simulink model "gm_UZ_EnDat"  (R2023b)
settings: Solver=FixedStepDiscrete  StartTime=0  StopTime=0.002  RelTol=1e-3
model workspace (MAT data in the model file):
  Select = 0
libraries: hdlsllib x314, hdlmdlgenlib x10, simulink x7, simulink_extras x3
(part 7 of 7)

== system gm_UZ_EnDat/UZ_ENDAT/ManualSerialize/padder/nibblepadding22/padding1 ==
  in : Inport  OutDataTypeStr=fixdt(0, 64, 0)  PortDimensions=1  SampleTime=1e-08
  Bit Shift2 : hdlsllib/Logic and Bit Operations/Bit Shift  mode=Shift Right Logical  N=double(1)
  Bit Slice2 : hdlsllib/Logic and Bit Operations/Bit Slice  lidx=double(0)  ridx=double(0)
  Data Type Conversion2 : DataTypeConversion  OutDataTypeStr=boolean  RndMeth=Nearest  SampleTime=1e-08  SaturateOnIntegerOverflow=off
  Switch2 : Switch  Criteria=u2 > Threshold  Threshold=double(0)  OutDataTypeStr=fixdt(0, 64, 0)  SampleTime=1e-08  SaturateOnIntegerOverflow=off  InputSameDT=off
  out : Outport  SampleTime=1e-08
  wires:
  Switch2/1 -> out/1
  Data Type Conversion2/1 -> Switch2/2
  Bit Slice2/1 -> Data Type Conversion2/1
  Bit Shift2/1 -> Switch2/3
  in/1 -> Bit Shift2/1, Bit Slice2/1, Switch2/1

== system gm_UZ_EnDat/UZ_ENDAT/ManualSerialize/padder/nibblepadding22/padding2 ==
  in : Inport  OutDataTypeStr=fixdt(0, 64, 0)  PortDimensions=1  SampleTime=1e-08
  Bit Shift2 : hdlsllib/Logic and Bit Operations/Bit Shift  mode=Shift Right Logical  N=double(1)
  Bit Slice2 : hdlsllib/Logic and Bit Operations/Bit Slice  lidx=double(0)  ridx=double(0)
  Data Type Conversion2 : DataTypeConversion  OutDataTypeStr=boolean  RndMeth=Nearest  SampleTime=1e-08  SaturateOnIntegerOverflow=off
  Switch2 : Switch  Criteria=u2 > Threshold  Threshold=double(0)  OutDataTypeStr=fixdt(0, 64, 0)  SampleTime=1e-08  SaturateOnIntegerOverflow=off  InputSameDT=off
  out : Outport  SampleTime=1e-08
  wires:
  in/1 -> Switch2/1, Bit Slice2/1, Bit Shift2/1
  Bit Shift2/1 -> Switch2/3
  Bit Slice2/1 -> Data Type Conversion2/1
  Data Type Conversion2/1 -> Switch2/2
  Switch2/1 -> out/1

== system gm_UZ_EnDat/UZ_ENDAT/ManualSerialize/padder/nibblepadding22/padding3 ==
  in : Inport  OutDataTypeStr=fixdt(0, 64, 0)  PortDimensions=1  SampleTime=1e-08
  Bit Shift2 : hdlsllib/Logic and Bit Operations/Bit Shift  mode=Shift Right Logical  N=double(1)
  Bit Slice2 : hdlsllib/Logic and Bit Operations/Bit Slice  lidx=double(0)  ridx=double(0)
  Data Type Conversion2 : DataTypeConversion  OutDataTypeStr=boolean  RndMeth=Nearest  SampleTime=1e-08  SaturateOnIntegerOverflow=off
  Switch2 : Switch  Criteria=u2 > Threshold  Threshold=double(0)  OutDataTypeStr=fixdt(0, 64, 0)  SampleTime=1e-08  SaturateOnIntegerOverflow=off  InputSameDT=off
  out : Outport  SampleTime=1e-08
  wires:
  in/1 -> Switch2/1, Bit Slice2/1, Bit Shift2/1
  Bit Shift2/1 -> Switch2/3
  Bit Slice2/1 -> Data Type Conversion2/1
  Data Type Conversion2/1 -> Switch2/2
  Switch2/1 -> out/1

== system gm_UZ_EnDat/UZ_ENDAT/ManualSerialize/padder/nibblepadding23/padding1 ==
  in : Inport  OutDataTypeStr=fixdt(0, 64, 0)  PortDimensions=1  SampleTime=1e-08
  Bit Shift2 : hdlsllib/Logic and Bit Operations/Bit Shift  mode=Shift Right Logical  N=double(1)
  Bit Slice2 : hdlsllib/Logic and Bit Operations/Bit Slice  lidx=double(0)  ridx=double(0)
  Data Type Conversion2 : DataTypeConversion  OutDataTypeStr=boolean  RndMeth=Nearest  SampleTime=1e-08  SaturateOnIntegerOverflow=off
  Switch2 : Switch  Criteria=u2 > Threshold  Threshold=double(0)  OutDataTypeStr=fixdt(0, 64, 0)  SampleTime=1e-08  SaturateOnIntegerOverflow=off  InputSameDT=off
  out : Outport  SampleTime=1e-08
  wires:
  Switch2/1 -> out/1
  Data Type Conversion2/1 -> Switch2/2
  Bit Slice2/1 -> Data Type Conversion2/1
  Bit Shift2/1 -> Switch2/3
  in/1 -> Bit Shift2/1, Bit Slice2/1, Switch2/1

== system gm_UZ_EnDat/UZ_ENDAT/ManualSerialize/padder/nibblepadding23/padding2 ==
  in : Inport  OutDataTypeStr=fixdt(0, 64, 0)  PortDimensions=1  SampleTime=1e-08
  Bit Shift2 : hdlsllib/Logic and Bit Operations/Bit Shift  mode=Shift Right Logical  N=double(1)
  Bit Slice2 : hdlsllib/Logic and Bit Operations/Bit Slice  lidx=double(0)  ridx=double(0)
  Data Type Conversion2 : DataTypeConversion  OutDataTypeStr=boolean  RndMeth=Nearest  SampleTime=1e-08  SaturateOnIntegerOverflow=off
  Switch2 : Switch  Criteria=u2 > Threshold  Threshold=double(0)  OutDataTypeStr=fixdt(0, 64, 0)  SampleTime=1e-08  SaturateOnIntegerOverflow=off  InputSameDT=off
  out : Outport  SampleTime=1e-08
  wires:
  in/1 -> Switch2/1, Bit Slice2/1, Bit Shift2/1
  Bit Shift2/1 -> Switch2/3
  Bit Slice2/1 -> Data Type Conversion2/1
  Data Type Conversion2/1 -> Switch2/2
  Switch2/1 -> out/1

== system gm_UZ_EnDat/UZ_ENDAT/ManualSerialize/padder/nibblepadding23/padding3 ==
  in : Inport  OutDataTypeStr=fixdt(0, 64, 0)  PortDimensions=1  SampleTime=1e-08
  Bit Shift2 : hdlsllib/Logic and Bit Operations/Bit Shift  mode=Shift Right Logical  N=double(1)
  Bit Slice2 : hdlsllib/Logic and Bit Operations/Bit Slice  lidx=double(0)  ridx=double(0)
  Data Type Conversion2 : DataTypeConversion  OutDataTypeStr=boolean  RndMeth=Nearest  SampleTime=1e-08  SaturateOnIntegerOverflow=off
  Switch2 : Switch  Criteria=u2 > Threshold  Threshold=double(0)  OutDataTypeStr=fixdt(0, 64, 0)  SampleTime=1e-08  SaturateOnIntegerOverflow=off  InputSameDT=off
  out : Outport  SampleTime=1e-08
  wires:
  in/1 -> Switch2/1, Bit Slice2/1, Bit Shift2/1
  Bit Shift2/1 -> Switch2/3
  Bit Slice2/1 -> Data Type Conversion2/1
  Data Type Conversion2/1 -> Switch2/2
  Switch2/1 -> out/1

== system gm_UZ_EnDat/UZ_ENDAT/ManualSerialize/padder/nibblepadding24/padding1 ==
  in : Inport  OutDataTypeStr=fixdt(0, 64, 0)  PortDimensions=1  SampleTime=1e-08
  Bit Shift2 : hdlsllib/Logic and Bit Operations/Bit Shift  mode=Shift Right Logical  N=double(1)
  Bit Slice2 : hdlsllib/Logic and Bit Operations/Bit Slice  lidx=double(0)  ridx=double(0)
  Data Type Conversion2 : DataTypeConversion  OutDataTypeStr=boolean  RndMeth=Nearest  SampleTime=1e-08  SaturateOnIntegerOverflow=off
  Switch2 : Switch  Criteria=u2 > Threshold  Threshold=double(0)  OutDataTypeStr=fixdt(0, 64, 0)  SampleTime=1e-08  SaturateOnIntegerOverflow=off  InputSameDT=off
  out : Outport  SampleTime=1e-08
  wires:
  Switch2/1 -> out/1
  Data Type Conversion2/1 -> Switch2/2
  Bit Slice2/1 -> Data Type Conversion2/1
  Bit Shift2/1 -> Switch2/3
  in/1 -> Bit Shift2/1, Bit Slice2/1, Switch2/1

== system gm_UZ_EnDat/UZ_ENDAT/ManualSerialize/padder/nibblepadding24/padding2 ==
  in : Inport  OutDataTypeStr=fixdt(0, 64, 0)  PortDimensions=1  SampleTime=1e-08
  Bit Shift2 : hdlsllib/Logic and Bit Operations/Bit Shift  mode=Shift Right Logical  N=double(1)
  Bit Slice2 : hdlsllib/Logic and Bit Operations/Bit Slice  lidx=double(0)  ridx=double(0)
  Data Type Conversion2 : DataTypeConversion  OutDataTypeStr=boolean  RndMeth=Nearest  SampleTime=1e-08  SaturateOnIntegerOverflow=off
  Switch2 : Switch  Criteria=u2 > Threshold  Threshold=double(0)  OutDataTypeStr=fixdt(0, 64, 0)  SampleTime=1e-08  SaturateOnIntegerOverflow=off  InputSameDT=off
  out : Outport  SampleTime=1e-08
  wires:
  in/1 -> Switch2/1, Bit Slice2/1, Bit Shift2/1
  Bit Shift2/1 -> Switch2/3
  Bit Slice2/1 -> Data Type Conversion2/1
  Data Type Conversion2/1 -> Switch2/2
  Switch2/1 -> out/1

== system gm_UZ_EnDat/UZ_ENDAT/ManualSerialize/padder/nibblepadding24/padding3 ==
  in : Inport  OutDataTypeStr=fixdt(0, 64, 0)  PortDimensions=1  SampleTime=1e-08
  Bit Shift2 : hdlsllib/Logic and Bit Operations/Bit Shift  mode=Shift Right Logical  N=double(1)
  Bit Slice2 : hdlsllib/Logic and Bit Operations/Bit Slice  lidx=double(0)  ridx=double(0)
  Data Type Conversion2 : DataTypeConversion  OutDataTypeStr=boolean  RndMeth=Nearest  SampleTime=1e-08  SaturateOnIntegerOverflow=off
  Switch2 : Switch  Criteria=u2 > Threshold  Threshold=double(0)  OutDataTypeStr=fixdt(0, 64, 0)  SampleTime=1e-08  SaturateOnIntegerOverflow=off  InputSameDT=off
  out : Outport  SampleTime=1e-08
  wires:
  in/1 -> Switch2/1, Bit Slice2/1, Bit Shift2/1
  Bit Shift2/1 -> Switch2/3
  Bit Slice2/1 -> Data Type Conversion2/1
  Data Type Conversion2/1 -> Switch2/2
  Switch2/1 -> out/1

== system gm_UZ_EnDat/UZ_ENDAT/ManualSerialize/padder/nibblepadding25/padding1 ==
  in : Inport  OutDataTypeStr=fixdt(0, 64, 0)  PortDimensions=1  SampleTime=1e-08
  Bit Shift2 : hdlsllib/Logic and Bit Operations/Bit Shift  mode=Shift Right Logical  N=double(1)
  Bit Slice2 : hdlsllib/Logic and Bit Operations/Bit Slice  lidx=double(0)  ridx=double(0)
  Data Type Conversion2 : DataTypeConversion  OutDataTypeStr=boolean  RndMeth=Nearest  SampleTime=1e-08  SaturateOnIntegerOverflow=off
  Switch2 : Switch  Criteria=u2 > Threshold  Threshold=double(0)  OutDataTypeStr=fixdt(0, 64, 0)  SampleTime=1e-08  SaturateOnIntegerOverflow=off  InputSameDT=off
  out : Outport  SampleTime=1e-08
  wires:
  Switch2/1 -> out/1
  Data Type Conversion2/1 -> Switch2/2
  Bit Slice2/1 -> Data Type Conversion2/1
  Bit Shift2/1 -> Switch2/3
  in/1 -> Bit Shift2/1, Bit Slice2/1, Switch2/1

== system gm_UZ_EnDat/UZ_ENDAT/ManualSerialize/padder/nibblepadding25/padding2 ==
  in : Inport  OutDataTypeStr=fixdt(0, 64, 0)  PortDimensions=1  SampleTime=1e-08
  Bit Shift2 : hdlsllib/Logic and Bit Operations/Bit Shift  mode=Shift Right Logical  N=double(1)
  Bit Slice2 : hdlsllib/Logic and Bit Operations/Bit Slice  lidx=double(0)  ridx=double(0)
  Data Type Conversion2 : DataTypeConversion  OutDataTypeStr=boolean  RndMeth=Nearest  SampleTime=1e-08  SaturateOnIntegerOverflow=off
  Switch2 : Switch  Criteria=u2 > Threshold  Threshold=double(0)  OutDataTypeStr=fixdt(0, 64, 0)  SampleTime=1e-08  SaturateOnIntegerOverflow=off  InputSameDT=off
  out : Outport  SampleTime=1e-08
  wires:
  in/1 -> Switch2/1, Bit Slice2/1, Bit Shift2/1
  Bit Shift2/1 -> Switch2/3
  Bit Slice2/1 -> Data Type Conversion2/1
  Data Type Conversion2/1 -> Switch2/2
  Switch2/1 -> out/1

== system gm_UZ_EnDat/UZ_ENDAT/ManualSerialize/padder/nibblepadding25/padding3 ==
  in : Inport  OutDataTypeStr=fixdt(0, 64, 0)  PortDimensions=1  SampleTime=1e-08
  Bit Shift2 : hdlsllib/Logic and Bit Operations/Bit Shift  mode=Shift Right Logical  N=double(1)
  Bit Slice2 : hdlsllib/Logic and Bit Operations/Bit Slice  lidx=double(0)  ridx=double(0)
  Data Type Conversion2 : DataTypeConversion  OutDataTypeStr=boolean  RndMeth=Nearest  SampleTime=1e-08  SaturateOnIntegerOverflow=off
  Switch2 : Switch  Criteria=u2 > Threshold  Threshold=double(0)  OutDataTypeStr=fixdt(0, 64, 0)  SampleTime=1e-08  SaturateOnIntegerOverflow=off  InputSameDT=off
  out : Outport  SampleTime=1e-08
  wires:
  in/1 -> Switch2/1, Bit Slice2/1, Bit Shift2/1
  Bit Shift2/1 -> Switch2/3
  Bit Slice2/1 -> Data Type Conversion2/1
  Data Type Conversion2/1 -> Switch2/2
  Switch2/1 -> out/1

== system gm_UZ_EnDat/UZ_ENDAT/ManualSerialize/padder/nibblepadding26/padding1 ==
  in : Inport  OutDataTypeStr=fixdt(0, 64, 0)  PortDimensions=1  SampleTime=1e-08
  Bit Shift2 : hdlsllib/Logic and Bit Operations/Bit Shift  mode=Shift Right Logical  N=double(1)
  Bit Slice2 : hdlsllib/Logic and Bit Operations/Bit Slice  lidx=double(0)  ridx=double(0)
  Data Type Conversion2 : DataTypeConversion  OutDataTypeStr=boolean  RndMeth=Nearest  SampleTime=1e-08  SaturateOnIntegerOverflow=off
  Switch2 : Switch  Criteria=u2 > Threshold  Threshold=double(0)  OutDataTypeStr=fixdt(0, 64, 0)  SampleTime=1e-08  SaturateOnIntegerOverflow=off  InputSameDT=off
  out : Outport  SampleTime=1e-08
  wires:
  Switch2/1 -> out/1
  Data Type Conversion2/1 -> Switch2/2
  Bit Slice2/1 -> Data Type Conversion2/1
  Bit Shift2/1 -> Switch2/3
  in/1 -> Bit Shift2/1, Bit Slice2/1, Switch2/1

== system gm_UZ_EnDat/UZ_ENDAT/ManualSerialize/padder/nibblepadding26/padding2 ==
  in : Inport  OutDataTypeStr=fixdt(0, 64, 0)  PortDimensions=1  SampleTime=1e-08
  Bit Shift2 : hdlsllib/Logic and Bit Operations/Bit Shift  mode=Shift Right Logical  N=double(1)
  Bit Slice2 : hdlsllib/Logic and Bit Operations/Bit Slice  lidx=double(0)  ridx=double(0)
  Data Type Conversion2 : DataTypeConversion  OutDataTypeStr=boolean  RndMeth=Nearest  SampleTime=1e-08  SaturateOnIntegerOverflow=off
  Switch2 : Switch  Criteria=u2 > Threshold  Threshold=double(0)  OutDataTypeStr=fixdt(0, 64, 0)  SampleTime=1e-08  SaturateOnIntegerOverflow=off  InputSameDT=off
  out : Outport  SampleTime=1e-08
  wires:
  in/1 -> Switch2/1, Bit Slice2/1, Bit Shift2/1
  Bit Shift2/1 -> Switch2/3
  Bit Slice2/1 -> Data Type Conversion2/1
  Data Type Conversion2/1 -> Switch2/2
  Switch2/1 -> out/1

== system gm_UZ_EnDat/UZ_ENDAT/ManualSerialize/padder/nibblepadding26/padding3 ==
  in : Inport  OutDataTypeStr=fixdt(0, 64, 0)  PortDimensions=1  SampleTime=1e-08
  Bit Shift2 : hdlsllib/Logic and Bit Operations/Bit Shift  mode=Shift Right Logical  N=double(1)
  Bit Slice2 : hdlsllib/Logic and Bit Operations/Bit Slice  lidx=double(0)  ridx=double(0)
  Data Type Conversion2 : DataTypeConversion  OutDataTypeStr=boolean  RndMeth=Nearest  SampleTime=1e-08  SaturateOnIntegerOverflow=off
  Switch2 : Switch  Criteria=u2 > Threshold  Threshold=double(0)  OutDataTypeStr=fixdt(0, 64, 0)  SampleTime=1e-08  SaturateOnIntegerOverflow=off  InputSameDT=off
  out : Outport  SampleTime=1e-08
  wires:
  in/1 -> Switch2/1, Bit Slice2/1, Bit Shift2/1
  Bit Shift2/1 -> Switch2/3
  Bit Slice2/1 -> Data Type Conversion2/1
  Data Type Conversion2/1 -> Switch2/2
  Switch2/1 -> out/1

== system gm_UZ_EnDat/UZ_ENDAT/ManualSerialize/padder/nibblepadding27/padding1 ==
  in : Inport  OutDataTypeStr=fixdt(0, 64, 0)  PortDimensions=1  SampleTime=1e-08
  Bit Shift2 : hdlsllib/Logic and Bit Operations/Bit Shift  mode=Shift Right Logical  N=double(1)
  Bit Slice2 : hdlsllib/Logic and Bit Operations/Bit Slice  lidx=double(0)  ridx=double(0)
  Data Type Conversion2 : DataTypeConversion  OutDataTypeStr=boolean  RndMeth=Nearest  SampleTime=1e-08  SaturateOnIntegerOverflow=off
  Switch2 : Switch  Criteria=u2 > Threshold  Threshold=double(0)  OutDataTypeStr=fixdt(0, 64, 0)  SampleTime=1e-08  SaturateOnIntegerOverflow=off  InputSameDT=off
  out : Outport  SampleTime=1e-08
  wires:
  Switch2/1 -> out/1
  Data Type Conversion2/1 -> Switch2/2
  Bit Slice2/1 -> Data Type Conversion2/1
  Bit Shift2/1 -> Switch2/3
  in/1 -> Bit Shift2/1, Bit Slice2/1, Switch2/1

== system gm_UZ_EnDat/UZ_ENDAT/ManualSerialize/padder/nibblepadding27/padding2 ==
  in : Inport  OutDataTypeStr=fixdt(0, 64, 0)  PortDimensions=1  SampleTime=1e-08
  Bit Shift2 : hdlsllib/Logic and Bit Operations/Bit Shift  mode=Shift Right Logical  N=double(1)
  Bit Slice2 : hdlsllib/Logic and Bit Operations/Bit Slice  lidx=double(0)  ridx=double(0)
  Data Type Conversion2 : DataTypeConversion  OutDataTypeStr=boolean  RndMeth=Nearest  SampleTime=1e-08  SaturateOnIntegerOverflow=off
  Switch2 : Switch  Criteria=u2 > Threshold  Threshold=double(0)  OutDataTypeStr=fixdt(0, 64, 0)  SampleTime=1e-08  SaturateOnIntegerOverflow=off  InputSameDT=off
  out : Outport  SampleTime=1e-08
  wires:
  in/1 -> Switch2/1, Bit Slice2/1, Bit Shift2/1
  Bit Shift2/1 -> Switch2/3
  Bit Slice2/1 -> Data Type Conversion2/1
  Data Type Conversion2/1 -> Switch2/2
  Switch2/1 -> out/1

== system gm_UZ_EnDat/UZ_ENDAT/ManualSerialize/padder/nibblepadding27/padding3 ==
  in : Inport  OutDataTypeStr=fixdt(0, 64, 0)  PortDimensions=1  SampleTime=1e-08
  Bit Shift2 : hdlsllib/Logic and Bit Operations/Bit Shift  mode=Shift Right Logical  N=double(1)
  Bit Slice2 : hdlsllib/Logic and Bit Operations/Bit Slice  lidx=double(0)  ridx=double(0)
  Data Type Conversion2 : DataTypeConversion  OutDataTypeStr=boolean  RndMeth=Nearest  SampleTime=1e-08  SaturateOnIntegerOverflow=off
  Switch2 : Switch  Criteria=u2 > Threshold  Threshold=double(0)  OutDataTypeStr=fixdt(0, 64, 0)  SampleTime=1e-08  SaturateOnIntegerOverflow=off  InputSameDT=off
  out : Outport  SampleTime=1e-08
  wires:
  in/1 -> Switch2/1, Bit Slice2/1, Bit Shift2/1
  Bit Shift2/1 -> Switch2/3
  Bit Slice2/1 -> Data Type Conversion2/1
  Data Type Conversion2/1 -> Switch2/2
  Switch2/1 -> out/1

== system gm_UZ_EnDat/UZ_ENDAT/ManualSerialize/padder/nibblepadding28/padding1 ==
  in : Inport  OutDataTypeStr=fixdt(0, 64, 0)  PortDimensions=1  SampleTime=1e-08
  Bit Shift2 : hdlsllib/Logic and Bit Operations/Bit Shift  mode=Shift Right Logical  N=double(1)
  Bit Slice2 : hdlsllib/Logic and Bit Operations/Bit Slice  lidx=double(0)  ridx=double(0)
  Data Type Conversion2 : DataTypeConversion  OutDataTypeStr=boolean  RndMeth=Nearest  SampleTime=1e-08  SaturateOnIntegerOverflow=off
  Switch2 : Switch  Criteria=u2 > Threshold  Threshold=double(0)  OutDataTypeStr=fixdt(0, 64, 0)  SampleTime=1e-08  SaturateOnIntegerOverflow=off  InputSameDT=off
  out : Outport  SampleTime=1e-08
  wires:
  Switch2/1 -> out/1
  Data Type Conversion2/1 -> Switch2/2
  Bit Slice2/1 -> Data Type Conversion2/1
  Bit Shift2/1 -> Switch2/3
  in/1 -> Bit Shift2/1, Bit Slice2/1, Switch2/1

== system gm_UZ_EnDat/UZ_ENDAT/ManualSerialize/padder/nibblepadding28/padding2 ==
  in : Inport  OutDataTypeStr=fixdt(0, 64, 0)  PortDimensions=1  SampleTime=1e-08
  Bit Shift2 : hdlsllib/Logic and Bit Operations/Bit Shift  mode=Shift Right Logical  N=double(1)
  Bit Slice2 : hdlsllib/Logic and Bit Operations/Bit Slice  lidx=double(0)  ridx=double(0)
  Data Type Conversion2 : DataTypeConversion  OutDataTypeStr=boolean  RndMeth=Nearest  SampleTime=1e-08  SaturateOnIntegerOverflow=off
  Switch2 : Switch  Criteria=u2 > Threshold  Threshold=double(0)  OutDataTypeStr=fixdt(0, 64, 0)  SampleTime=1e-08  SaturateOnIntegerOverflow=off  InputSameDT=off
  out : Outport  SampleTime=1e-08
  wires:
  in/1 -> Switch2/1, Bit Slice2/1, Bit Shift2/1
  Bit Shift2/1 -> Switch2/3
  Bit Slice2/1 -> Data Type Conversion2/1
  Data Type Conversion2/1 -> Switch2/2
  Switch2/1 -> out/1

== system gm_UZ_EnDat/UZ_ENDAT/ManualSerialize/padder/nibblepadding28/padding3 ==
  in : Inport  OutDataTypeStr=fixdt(0, 64, 0)  PortDimensions=1  SampleTime=1e-08
  Bit Shift2 : hdlsllib/Logic and Bit Operations/Bit Shift  mode=Shift Right Logical  N=double(1)
  Bit Slice2 : hdlsllib/Logic and Bit Operations/Bit Slice  lidx=double(0)  ridx=double(0)
  Data Type Conversion2 : DataTypeConversion  OutDataTypeStr=boolean  RndMeth=Nearest  SampleTime=1e-08  SaturateOnIntegerOverflow=off
  Switch2 : Switch  Criteria=u2 > Threshold  Threshold=double(0)  OutDataTypeStr=fixdt(0, 64, 0)  SampleTime=1e-08  SaturateOnIntegerOverflow=off  InputSameDT=off
  out : Outport  SampleTime=1e-08
  wires:
  in/1 -> Switch2/1, Bit Slice2/1, Bit Shift2/1
  Bit Shift2/1 -> Switch2/3
  Bit Slice2/1 -> Data Type Conversion2/1
  Data Type Conversion2/1 -> Switch2/2
  Switch2/1 -> out/1

== system gm_UZ_EnDat/UZ_ENDAT/ManualSerialize/padder/nibblepadding29/padding1 ==
  in : Inport  OutDataTypeStr=fixdt(0, 64, 0)  PortDimensions=1  SampleTime=1e-08
  Bit Shift2 : hdlsllib/Logic and Bit Operations/Bit Shift  mode=Shift Right Logical  N=double(1)
  Bit Slice2 : hdlsllib/Logic and Bit Operations/Bit Slice  lidx=double(0)  ridx=double(0)
  Data Type Conversion2 : DataTypeConversion  OutDataTypeStr=boolean  RndMeth=Nearest  SampleTime=1e-08  SaturateOnIntegerOverflow=off
  Switch2 : Switch  Criteria=u2 > Threshold  Threshold=double(0)  OutDataTypeStr=fixdt(0, 64, 0)  SampleTime=1e-08  SaturateOnIntegerOverflow=off  InputSameDT=off
  out : Outport  SampleTime=1e-08
  wires:
  Switch2/1 -> out/1
  Data Type Conversion2/1 -> Switch2/2
  Bit Slice2/1 -> Data Type Conversion2/1
  Bit Shift2/1 -> Switch2/3
  in/1 -> Bit Shift2/1, Bit Slice2/1, Switch2/1

== system gm_UZ_EnDat/UZ_ENDAT/ManualSerialize/padder/nibblepadding29/padding2 ==
  in : Inport  OutDataTypeStr=fixdt(0, 64, 0)  PortDimensions=1  SampleTime=1e-08
  Bit Shift2 : hdlsllib/Logic and Bit Operations/Bit Shift  mode=Shift Right Logical  N=double(1)
  Bit Slice2 : hdlsllib/Logic and Bit Operations/Bit Slice  lidx=double(0)  ridx=double(0)
  Data Type Conversion2 : DataTypeConversion  OutDataTypeStr=boolean  RndMeth=Nearest  SampleTime=1e-08  SaturateOnIntegerOverflow=off
  Switch2 : Switch  Criteria=u2 > Threshold  Threshold=double(0)  OutDataTypeStr=fixdt(0, 64, 0)  SampleTime=1e-08  SaturateOnIntegerOverflow=off  InputSameDT=off
  out : Outport  SampleTime=1e-08
  wires:
  in/1 -> Switch2/1, Bit Slice2/1, Bit Shift2/1
  Bit Shift2/1 -> Switch2/3
  Bit Slice2/1 -> Data Type Conversion2/1
  Data Type Conversion2/1 -> Switch2/2
  Switch2/1 -> out/1

== system gm_UZ_EnDat/UZ_ENDAT/ManualSerialize/padder/nibblepadding29/padding3 ==
  in : Inport  OutDataTypeStr=fixdt(0, 64, 0)  PortDimensions=1  SampleTime=1e-08
  Bit Shift2 : hdlsllib/Logic and Bit Operations/Bit Shift  mode=Shift Right Logical  N=double(1)
  Bit Slice2 : hdlsllib/Logic and Bit Operations/Bit Slice  lidx=double(0)  ridx=double(0)
  Data Type Conversion2 : DataTypeConversion  OutDataTypeStr=boolean  RndMeth=Nearest  SampleTime=1e-08  SaturateOnIntegerOverflow=off
  Switch2 : Switch  Criteria=u2 > Threshold  Threshold=double(0)  OutDataTypeStr=fixdt(0, 64, 0)  SampleTime=1e-08  SaturateOnIntegerOverflow=off  InputSameDT=off
  out : Outport  SampleTime=1e-08
  wires:
  in/1 -> Switch2/1, Bit Slice2/1, Bit Shift2/1
  Bit Shift2/1 -> Switch2/3
  Bit Slice2/1 -> Data Type Conversion2/1
  Data Type Conversion2/1 -> Switch2/2
  Switch2/1 -> out/1

== system gm_UZ_EnDat/UZ_ENDAT/ManualSerialize/padder/nibblepadding3/padding1 ==
  in : Inport  OutDataTypeStr=fixdt(0, 64, 0)  PortDimensions=1  SampleTime=1e-08
  Bit Shift2 : hdlsllib/Logic and Bit Operations/Bit Shift  mode=Shift Right Logical  N=double(1)
  Bit Slice2 : hdlsllib/Logic and Bit Operations/Bit Slice  lidx=double(0)  ridx=double(0)
  Data Type Conversion2 : DataTypeConversion  OutDataTypeStr=boolean  RndMeth=Nearest  SampleTime=1e-08  SaturateOnIntegerOverflow=off
  Switch2 : Switch  Criteria=u2 > Threshold  Threshold=double(0)  OutDataTypeStr=fixdt(0, 64, 0)  SampleTime=1e-08  SaturateOnIntegerOverflow=off  InputSameDT=off
  out : Outport  SampleTime=1e-08
  wires:
  Switch2/1 -> out/1
  Data Type Conversion2/1 -> Switch2/2
  Bit Slice2/1 -> Data Type Conversion2/1
  Bit Shift2/1 -> Switch2/3
  in/1 -> Bit Shift2/1, Bit Slice2/1, Switch2/1

== system gm_UZ_EnDat/UZ_ENDAT/ManualSerialize/padder/nibblepadding3/padding2 ==
  in : Inport  OutDataTypeStr=fixdt(0, 64, 0)  PortDimensions=1  SampleTime=1e-08
  Bit Shift2 : hdlsllib/Logic and Bit Operations/Bit Shift  mode=Shift Right Logical  N=double(1)
  Bit Slice2 : hdlsllib/Logic and Bit Operations/Bit Slice  lidx=double(0)  ridx=double(0)
  Data Type Conversion2 : DataTypeConversion  OutDataTypeStr=boolean  RndMeth=Nearest  SampleTime=1e-08  SaturateOnIntegerOverflow=off
  Switch2 : Switch  Criteria=u2 > Threshold  Threshold=double(0)  OutDataTypeStr=fixdt(0, 64, 0)  SampleTime=1e-08  SaturateOnIntegerOverflow=off  InputSameDT=off
  out : Outport  SampleTime=1e-08
  wires:
  in/1 -> Switch2/1, Bit Slice2/1, Bit Shift2/1
  Bit Shift2/1 -> Switch2/3
  Bit Slice2/1 -> Data Type Conversion2/1
  Data Type Conversion2/1 -> Switch2/2
  Switch2/1 -> out/1

== system gm_UZ_EnDat/UZ_ENDAT/ManualSerialize/padder/nibblepadding3/padding3 ==
  in : Inport  OutDataTypeStr=fixdt(0, 64, 0)  PortDimensions=1  SampleTime=1e-08
  Bit Shift2 : hdlsllib/Logic and Bit Operations/Bit Shift  mode=Shift Right Logical  N=double(1)
  Bit Slice2 : hdlsllib/Logic and Bit Operations/Bit Slice  lidx=double(0)  ridx=double(0)
  Data Type Conversion2 : DataTypeConversion  OutDataTypeStr=boolean  RndMeth=Nearest  SampleTime=1e-08  SaturateOnIntegerOverflow=off
  Switch2 : Switch  Criteria=u2 > Threshold  Threshold=double(0)  OutDataTypeStr=fixdt(0, 64, 0)  SampleTime=1e-08  SaturateOnIntegerOverflow=off  InputSameDT=off
  out : Outport  SampleTime=1e-08
  wires:
  in/1 -> Switch2/1, Bit Slice2/1, Bit Shift2/1
  Bit Shift2/1 -> Switch2/3
  Bit Slice2/1 -> Data Type Conversion2/1
  Data Type Conversion2/1 -> Switch2/2
  Switch2/1 -> out/1

== system gm_UZ_EnDat/UZ_ENDAT/ManualSerialize/padder/nibblepadding30/padding1 ==
  in : Inport  OutDataTypeStr=fixdt(0, 64, 0)  PortDimensions=1  SampleTime=1e-08
  Bit Shift2 : hdlsllib/Logic and Bit Operations/Bit Shift  mode=Shift Right Logical  N=double(1)
  Bit Slice2 : hdlsllib/Logic and Bit Operations/Bit Slice  lidx=double(0)  ridx=double(0)
  Data Type Conversion2 : DataTypeConversion  OutDataTypeStr=boolean  RndMeth=Nearest  SampleTime=1e-08  SaturateOnIntegerOverflow=off
  Switch2 : Switch  Criteria=u2 > Threshold  Threshold=double(0)  OutDataTypeStr=fixdt(0, 64, 0)  SampleTime=1e-08  SaturateOnIntegerOverflow=off  InputSameDT=off
  out : Outport  SampleTime=1e-08
  wires:
  Switch2/1 -> out/1
  Data Type Conversion2/1 -> Switch2/2
  Bit Slice2/1 -> Data Type Conversion2/1
  Bit Shift2/1 -> Switch2/3
  in/1 -> Bit Shift2/1, Bit Slice2/1, Switch2/1

== system gm_UZ_EnDat/UZ_ENDAT/ManualSerialize/padder/nibblepadding30/padding2 ==
  in : Inport  OutDataTypeStr=fixdt(0, 64, 0)  PortDimensions=1  SampleTime=1e-08
  Bit Shift2 : hdlsllib/Logic and Bit Operations/Bit Shift  mode=Shift Right Logical  N=double(1)
  Bit Slice2 : hdlsllib/Logic and Bit Operations/Bit Slice  lidx=double(0)  ridx=double(0)
  Data Type Conversion2 : DataTypeConversion  OutDataTypeStr=boolean  RndMeth=Nearest  SampleTime=1e-08  SaturateOnIntegerOverflow=off
  Switch2 : Switch  Criteria=u2 > Threshold  Threshold=double(0)  OutDataTypeStr=fixdt(0, 64, 0)  SampleTime=1e-08  SaturateOnIntegerOverflow=off  InputSameDT=off
  out : Outport  SampleTime=1e-08
  wires:
  in/1 -> Switch2/1, Bit Slice2/1, Bit Shift2/1
  Bit Shift2/1 -> Switch2/3
  Bit Slice2/1 -> Data Type Conversion2/1
  Data Type Conversion2/1 -> Switch2/2
  Switch2/1 -> out/1

== system gm_UZ_EnDat/UZ_ENDAT/ManualSerialize/padder/nibblepadding30/padding3 ==
  in : Inport  OutDataTypeStr=fixdt(0, 64, 0)  PortDimensions=1  SampleTime=1e-08
  Bit Shift2 : hdlsllib/Logic and Bit Operations/Bit Shift  mode=Shift Right Logical  N=double(1)
  Bit Slice2 : hdlsllib/Logic and Bit Operations/Bit Slice  lidx=double(0)  ridx=double(0)
  Data Type Conversion2 : DataTypeConversion  OutDataTypeStr=boolean  RndMeth=Nearest  SampleTime=1e-08  SaturateOnIntegerOverflow=off
  Switch2 : Switch  Criteria=u2 > Threshold  Threshold=double(0)  OutDataTypeStr=fixdt(0, 64, 0)  SampleTime=1e-08  SaturateOnIntegerOverflow=off  InputSameDT=off
  out : Outport  SampleTime=1e-08
  wires:
  in/1 -> Switch2/1, Bit Slice2/1, Bit Shift2/1
  Bit Shift2/1 -> Switch2/3
  Bit Slice2/1 -> Data Type Conversion2/1
  Data Type Conversion2/1 -> Switch2/2
  Switch2/1 -> out/1

== system gm_UZ_EnDat/UZ_ENDAT/ManualSerialize/padder/nibblepadding4/padding1 ==
  in : Inport  OutDataTypeStr=fixdt(0, 64, 0)  PortDimensions=1  SampleTime=1e-08
  Bit Shift2 : hdlsllib/Logic and Bit Operations/Bit Shift  mode=Shift Right Logical  N=double(1)
  Bit Slice2 : hdlsllib/Logic and Bit Operations/Bit Slice  lidx=double(0)  ridx=double(0)
  Data Type Conversion2 : DataTypeConversion  OutDataTypeStr=boolean  RndMeth=Nearest  SampleTime=1e-08  SaturateOnIntegerOverflow=off
  Switch2 : Switch  Criteria=u2 > Threshold  Threshold=double(0)  OutDataTypeStr=fixdt(0, 64, 0)  SampleTime=1e-08  SaturateOnIntegerOverflow=off  InputSameDT=off
  out : Outport  SampleTime=1e-08
  wires:
  Switch2/1 -> out/1
  Data Type Conversion2/1 -> Switch2/2
  Bit Slice2/1 -> Data Type Conversion2/1
  Bit Shift2/1 -> Switch2/3
  in/1 -> Bit Shift2/1, Bit Slice2/1, Switch2/1

== system gm_UZ_EnDat/UZ_ENDAT/ManualSerialize/padder/nibblepadding4/padding2 ==
  in : Inport  OutDataTypeStr=fixdt(0, 64, 0)  PortDimensions=1  SampleTime=1e-08
  Bit Shift2 : hdlsllib/Logic and Bit Operations/Bit Shift  mode=Shift Right Logical  N=double(1)
  Bit Slice2 : hdlsllib/Logic and Bit Operations/Bit Slice  lidx=double(0)  ridx=double(0)
  Data Type Conversion2 : DataTypeConversion  OutDataTypeStr=boolean  RndMeth=Nearest  SampleTime=1e-08  SaturateOnIntegerOverflow=off
  Switch2 : Switch  Criteria=u2 > Threshold  Threshold=double(0)  OutDataTypeStr=fixdt(0, 64, 0)  SampleTime=1e-08  SaturateOnIntegerOverflow=off  InputSameDT=off
  out : Outport  SampleTime=1e-08
  wires:
  in/1 -> Switch2/1, Bit Slice2/1, Bit Shift2/1
  Bit Shift2/1 -> Switch2/3
  Bit Slice2/1 -> Data Type Conversion2/1
  Data Type Conversion2/1 -> Switch2/2
  Switch2/1 -> out/1

== system gm_UZ_EnDat/UZ_ENDAT/ManualSerialize/padder/nibblepadding4/padding3 ==
  in : Inport  OutDataTypeStr=fixdt(0, 64, 0)  PortDimensions=1  SampleTime=1e-08
  Bit Shift2 : hdlsllib/Logic and Bit Operations/Bit Shift  mode=Shift Right Logical  N=double(1)
  Bit Slice2 : hdlsllib/Logic and Bit Operations/Bit Slice  lidx=double(0)  ridx=double(0)
  Data Type Conversion2 : DataTypeConversion  OutDataTypeStr=boolean  RndMeth=Nearest  SampleTime=1e-08  SaturateOnIntegerOverflow=off
  Switch2 : Switch  Criteria=u2 > Threshold  Threshold=double(0)  OutDataTypeStr=fixdt(0, 64, 0)  SampleTime=1e-08  SaturateOnIntegerOverflow=off  InputSameDT=off
  out : Outport  SampleTime=1e-08
  wires:
  in/1 -> Switch2/1, Bit Slice2/1, Bit Shift2/1
  Bit Shift2/1 -> Switch2/3
  Bit Slice2/1 -> Data Type Conversion2/1
  Data Type Conversion2/1 -> Switch2/2
  Switch2/1 -> out/1

== system gm_UZ_EnDat/UZ_ENDAT/ManualSerialize/padder/nibblepadding6/padding1 ==
  in : Inport  OutDataTypeStr=fixdt(0, 64, 0)  PortDimensions=1  SampleTime=1e-08
  Bit Shift2 : hdlsllib/Logic and Bit Operations/Bit Shift  mode=Shift Right Logical  N=double(1)
  Bit Slice2 : hdlsllib/Logic and Bit Operations/Bit Slice  lidx=double(0)  ridx=double(0)
  Data Type Conversion2 : DataTypeConversion  OutDataTypeStr=boolean  RndMeth=Nearest  SampleTime=1e-08  SaturateOnIntegerOverflow=off
  Switch2 : Switch  Criteria=u2 > Threshold  Threshold=double(0)  OutDataTypeStr=fixdt(0, 64, 0)  SampleTime=1e-08  SaturateOnIntegerOverflow=off  InputSameDT=off
  out : Outport  SampleTime=1e-08
  wires:
  Switch2/1 -> out/1
  Data Type Conversion2/1 -> Switch2/2
  Bit Slice2/1 -> Data Type Conversion2/1
  Bit Shift2/1 -> Switch2/3
  in/1 -> Bit Shift2/1, Bit Slice2/1, Switch2/1

== system gm_UZ_EnDat/UZ_ENDAT/ManualSerialize/padder/nibblepadding6/padding2 ==
  in : Inport  OutDataTypeStr=fixdt(0, 64, 0)  PortDimensions=1  SampleTime=1e-08
  Bit Shift2 : hdlsllib/Logic and Bit Operations/Bit Shift  mode=Shift Right Logical  N=double(1)
  Bit Slice2 : hdlsllib/Logic and Bit Operations/Bit Slice  lidx=double(0)  ridx=double(0)
  Data Type Conversion2 : DataTypeConversion  OutDataTypeStr=boolean  RndMeth=Nearest  SampleTime=1e-08  SaturateOnIntegerOverflow=off
  Switch2 : Switch  Criteria=u2 > Threshold  Threshold=double(0)  OutDataTypeStr=fixdt(0, 64, 0)  SampleTime=1e-08  SaturateOnIntegerOverflow=off  InputSameDT=off
  out : Outport  SampleTime=1e-08
  wires:
  in/1 -> Switch2/1, Bit Slice2/1, Bit Shift2/1
  Bit Shift2/1 -> Switch2/3
  Bit Slice2/1 -> Data Type Conversion2/1
  Data Type Conversion2/1 -> Switch2/2
  Switch2/1 -> out/1

== system gm_UZ_EnDat/UZ_ENDAT/ManualSerialize/padder/nibblepadding6/padding3 ==
  in : Inport  OutDataTypeStr=fixdt(0, 64, 0)  PortDimensions=1  SampleTime=1e-08
  Bit Shift2 : hdlsllib/Logic and Bit Operations/Bit Shift  mode=Shift Right Logical  N=double(1)
  Bit Slice2 : hdlsllib/Logic and Bit Operations/Bit Slice  lidx=double(0)  ridx=double(0)
  Data Type Conversion2 : DataTypeConversion  OutDataTypeStr=boolean  RndMeth=Nearest  SampleTime=1e-08  SaturateOnIntegerOverflow=off
  Switch2 : Switch  Criteria=u2 > Threshold  Threshold=double(0)  OutDataTypeStr=fixdt(0, 64, 0)  SampleTime=1e-08  SaturateOnIntegerOverflow=off  InputSameDT=off
  out : Outport  SampleTime=1e-08
  wires:
  in/1 -> Switch2/1, Bit Slice2/1, Bit Shift2/1
  Bit Shift2/1 -> Switch2/3
  Bit Slice2/1 -> Data Type Conversion2/1
  Data Type Conversion2/1 -> Switch2/2
  Switch2/1 -> out/1

== system gm_UZ_EnDat/UZ_ENDAT/ManualSerialize/padder/nibblepadding7/padding1 ==
  in : Inport  OutDataTypeStr=fixdt(0, 64, 0)  PortDimensions=1  SampleTime=1e-08
  Bit Shift2 : hdlsllib/Logic and Bit Operations/Bit Shift  mode=Shift Right Logical  N=double(1)
  Bit Slice2 : hdlsllib/Logic and Bit Operations/Bit Slice  lidx=double(0)  ridx=double(0)
  Data Type Conversion2 : DataTypeConversion  OutDataTypeStr=boolean  RndMeth=Nearest  SampleTime=1e-08  SaturateOnIntegerOverflow=off
  Switch2 : Switch  Criteria=u2 > Threshold  Threshold=double(0)  OutDataTypeStr=fixdt(0, 64, 0)  SampleTime=1e-08  SaturateOnIntegerOverflow=off  InputSameDT=off
  out : Outport  SampleTime=1e-08
  wires:
  Switch2/1 -> out/1
  Data Type Conversion2/1 -> Switch2/2
  Bit Slice2/1 -> Data Type Conversion2/1
  Bit Shift2/1 -> Switch2/3
  in/1 -> Bit Shift2/1, Bit Slice2/1, Switch2/1

== system gm_UZ_EnDat/UZ_ENDAT/ManualSerialize/padder/nibblepadding7/padding2 ==
  in : Inport  OutDataTypeStr=fixdt(0, 64, 0)  PortDimensions=1  SampleTime=1e-08
  Bit Shift2 : hdlsllib/Logic and Bit Operations/Bit Shift  mode=Shift Right Logical  N=double(1)
  Bit Slice2 : hdlsllib/Logic and Bit Operations/Bit Slice  lidx=double(0)  ridx=double(0)
  Data Type Conversion2 : DataTypeConversion  OutDataTypeStr=boolean  RndMeth=Nearest  SampleTime=1e-08  SaturateOnIntegerOverflow=off
  Switch2 : Switch  Criteria=u2 > Threshold  Threshold=double(0)  OutDataTypeStr=fixdt(0, 64, 0)  SampleTime=1e-08  SaturateOnIntegerOverflow=off  InputSameDT=off
  out : Outport  SampleTime=1e-08
  wires:
  in/1 -> Switch2/1, Bit Slice2/1, Bit Shift2/1
  Bit Shift2/1 -> Switch2/3
  Bit Slice2/1 -> Data Type Conversion2/1
  Data Type Conversion2/1 -> Switch2/2
  Switch2/1 -> out/1

== system gm_UZ_EnDat/UZ_ENDAT/ManualSerialize/padder/nibblepadding7/padding3 ==
  in : Inport  OutDataTypeStr=fixdt(0, 64, 0)  PortDimensions=1  SampleTime=1e-08
  Bit Shift2 : hdlsllib/Logic and Bit Operations/Bit Shift  mode=Shift Right Logical  N=double(1)
  Bit Slice2 : hdlsllib/Logic and Bit Operations/Bit Slice  lidx=double(0)  ridx=double(0)
  Data Type Conversion2 : DataTypeConversion  OutDataTypeStr=boolean  RndMeth=Nearest  SampleTime=1e-08  SaturateOnIntegerOverflow=off
  Switch2 : Switch  Criteria=u2 > Threshold  Threshold=double(0)  OutDataTypeStr=fixdt(0, 64, 0)  SampleTime=1e-08  SaturateOnIntegerOverflow=off  InputSameDT=off
  out : Outport  SampleTime=1e-08
  wires:
  in/1 -> Switch2/1, Bit Slice2/1, Bit Shift2/1
  Bit Shift2/1 -> Switch2/3
  Bit Slice2/1 -> Data Type Conversion2/1
  Data Type Conversion2/1 -> Switch2/2
  Switch2/1 -> out/1

== system gm_UZ_EnDat/UZ_ENDAT/ManualSerialize/padder/nibblepadding8/padding1 ==
  in : Inport  OutDataTypeStr=fixdt(0, 64, 0)  PortDimensions=1  SampleTime=1e-08
  Bit Shift2 : hdlsllib/Logic and Bit Operations/Bit Shift  mode=Shift Right Logical  N=double(1)
  Bit Slice2 : hdlsllib/Logic and Bit Operations/Bit Slice  lidx=double(0)  ridx=double(0)
  Data Type Conversion2 : DataTypeConversion  OutDataTypeStr=boolean  RndMeth=Nearest  SampleTime=1e-08  SaturateOnIntegerOverflow=off
  Switch2 : Switch  Criteria=u2 > Threshold  Threshold=double(0)  OutDataTypeStr=fixdt(0, 64, 0)  SampleTime=1e-08  SaturateOnIntegerOverflow=off  InputSameDT=off
  out : Outport  SampleTime=1e-08
  wires:
  Switch2/1 -> out/1
  Data Type Conversion2/1 -> Switch2/2
  Bit Slice2/1 -> Data Type Conversion2/1
  Bit Shift2/1 -> Switch2/3
  in/1 -> Bit Shift2/1, Bit Slice2/1, Switch2/1

== system gm_UZ_EnDat/UZ_ENDAT/ManualSerialize/padder/nibblepadding8/padding2 ==
  in : Inport  OutDataTypeStr=fixdt(0, 64, 0)  PortDimensions=1  SampleTime=1e-08
  Bit Shift2 : hdlsllib/Logic and Bit Operations/Bit Shift  mode=Shift Right Logical  N=double(1)
  Bit Slice2 : hdlsllib/Logic and Bit Operations/Bit Slice  lidx=double(0)  ridx=double(0)
  Data Type Conversion2 : DataTypeConversion  OutDataTypeStr=boolean  RndMeth=Nearest  SampleTime=1e-08  SaturateOnIntegerOverflow=off
  Switch2 : Switch  Criteria=u2 > Threshold  Threshold=double(0)  OutDataTypeStr=fixdt(0, 64, 0)  SampleTime=1e-08  SaturateOnIntegerOverflow=off  InputSameDT=off
  out : Outport  SampleTime=1e-08
  wires:
  in/1 -> Switch2/1, Bit Slice2/1, Bit Shift2/1
  Bit Shift2/1 -> Switch2/3
  Bit Slice2/1 -> Data Type Conversion2/1
  Data Type Conversion2/1 -> Switch2/2
  Switch2/1 -> out/1

== system gm_UZ_EnDat/UZ_ENDAT/ManualSerialize/padder/nibblepadding8/padding3 ==
  in : Inport  OutDataTypeStr=fixdt(0, 64, 0)  PortDimensions=1  SampleTime=1e-08
  Bit Shift2 : hdlsllib/Logic and Bit Operations/Bit Shift  mode=Shift Right Logical  N=double(1)
  Bit Slice2 : hdlsllib/Logic and Bit Operations/Bit Slice  lidx=double(0)  ridx=double(0)
  Data Type Conversion2 : DataTypeConversion  OutDataTypeStr=boolean  RndMeth=Nearest  SampleTime=1e-08  SaturateOnIntegerOverflow=off
  Switch2 : Switch  Criteria=u2 > Threshold  Threshold=double(0)  OutDataTypeStr=fixdt(0, 64, 0)  SampleTime=1e-08  SaturateOnIntegerOverflow=off  InputSameDT=off
  out : Outport  SampleTime=1e-08
  wires:
  in/1 -> Switch2/1, Bit Slice2/1, Bit Shift2/1
  Bit Shift2/1 -> Switch2/3
  Bit Slice2/1 -> Data Type Conversion2/1
  Data Type Conversion2/1 -> Switch2/2
  Switch2/1 -> out/1

== system gm_UZ_EnDat/UZ_ENDAT/ManualSerialize/padder/nibblepadding9/padding1 ==
  in : Inport  OutDataTypeStr=fixdt(0, 64, 0)  PortDimensions=1  SampleTime=1e-08
  Bit Shift2 : hdlsllib/Logic and Bit Operations/Bit Shift  mode=Shift Right Logical  N=double(1)
  Bit Slice2 : hdlsllib/Logic and Bit Operations/Bit Slice  lidx=double(0)  ridx=double(0)
  Data Type Conversion2 : DataTypeConversion  OutDataTypeStr=boolean  RndMeth=Nearest  SampleTime=1e-08  SaturateOnIntegerOverflow=off
  Switch2 : Switch  Criteria=u2 > Threshold  Threshold=double(0)  OutDataTypeStr=fixdt(0, 64, 0)  SampleTime=1e-08  SaturateOnIntegerOverflow=off  InputSameDT=off
  out : Outport  SampleTime=1e-08
  wires:
  Switch2/1 -> out/1
  Data Type Conversion2/1 -> Switch2/2
  Bit Slice2/1 -> Data Type Conversion2/1
  Bit Shift2/1 -> Switch2/3
  in/1 -> Bit Shift2/1, Bit Slice2/1, Switch2/1

== system gm_UZ_EnDat/UZ_ENDAT/ManualSerialize/padder/nibblepadding9/padding2 ==
  in : Inport  OutDataTypeStr=fixdt(0, 64, 0)  PortDimensions=1  SampleTime=1e-08
  Bit Shift2 : hdlsllib/Logic and Bit Operations/Bit Shift  mode=Shift Right Logical  N=double(1)
  Bit Slice2 : hdlsllib/Logic and Bit Operations/Bit Slice  lidx=double(0)  ridx=double(0)
  Data Type Conversion2 : DataTypeConversion  OutDataTypeStr=boolean  RndMeth=Nearest  SampleTime=1e-08  SaturateOnIntegerOverflow=off
  Switch2 : Switch  Criteria=u2 > Threshold  Threshold=double(0)  OutDataTypeStr=fixdt(0, 64, 0)  SampleTime=1e-08  SaturateOnIntegerOverflow=off  InputSameDT=off
  out : Outport  SampleTime=1e-08
  wires:
  in/1 -> Switch2/1, Bit Slice2/1, Bit Shift2/1
  Bit Shift2/1 -> Switch2/3
  Bit Slice2/1 -> Data Type Conversion2/1
  Data Type Conversion2/1 -> Switch2/2
  Switch2/1 -> out/1

== system gm_UZ_EnDat/UZ_ENDAT/ManualSerialize/padder/nibblepadding9/padding3 ==
  in : Inport  OutDataTypeStr=fixdt(0, 64, 0)  PortDimensions=1  SampleTime=1e-08
  Bit Shift2 : hdlsllib/Logic and Bit Operations/Bit Shift  mode=Shift Right Logical  N=double(1)
  Bit Slice2 : hdlsllib/Logic and Bit Operations/Bit Slice  lidx=double(0)  ridx=double(0)
  Data Type Conversion2 : DataTypeConversion  OutDataTypeStr=boolean  RndMeth=Nearest  SampleTime=1e-08  SaturateOnIntegerOverflow=off
  Switch2 : Switch  Criteria=u2 > Threshold  Threshold=double(0)  OutDataTypeStr=fixdt(0, 64, 0)  SampleTime=1e-08  SaturateOnIntegerOverflow=off  InputSameDT=off
  out : Outport  SampleTime=1e-08
  wires:
  in/1 -> Switch2/1, Bit Slice2/1, Bit Shift2/1
  Bit Shift2/1 -> Switch2/3
  Bit Slice2/1 -> Data Type Conversion2/1
  Data Type Conversion2/1 -> Switch2/2
  Switch2/1 -> out/1

== system gm_UZ_EnDat/UZ_ENDAT/Subsystem2/ManualDeserializere/ramwatcher/Increment Stored Integer ==
  u : Inport  OutDataTypeStr=uint16
  FixPt Constant : Constant  OutDataTypeStr=uint16  SampleTime=-1
  FixPt Data Type Duplicate : DataTypeDuplicate  DisableCoverage=on  NumInputPorts=3
  FixPt Gateway In : DataTypeConversion  OutDataTypeStr=fixdt(0,16,0)
  FixPt Sum1 : Sum  OutDataTypeStr=uint16  AccumDataTypeStr=uint16
  sigspec : SignalSpecification  OutDataTypeStr=uint16  Dimensions=1
  y : Outport  InitialOutput=0
  wires:
  u/1 -> FixPt Sum1/1, FixPt Data Type Duplicate/2
  FixPt Constant/1 -> sigspec/1
  FixPt Gateway In/1 -> FixPt Sum1/2, FixPt Data Type Duplicate/3
  FixPt Sum1/1 -> FixPt Data Type Duplicate/1, y/1
  sigspec/1 -> FixPt Gateway In/1

== system gm_UZ_EnDat/UZ_ENDAT/timingprovider/CLKCNTER_POSCNTR/Positional_Counter/Increment Stored Integer ==
  u : Inport  OutDataTypeStr=uint32
  FixPt Constant : Constant  OutDataTypeStr=uint32  SampleTime=-1
  FixPt Data Type Duplicate : DataTypeDuplicate  DisableCoverage=on  NumInputPorts=3
  FixPt Gateway In : DataTypeConversion  OutDataTypeStr=fixdt(0,32,0)
  FixPt Sum1 : Sum  OutDataTypeStr=uint32  AccumDataTypeStr=uint32
  sigspec : SignalSpecification  OutDataTypeStr=uint32  Dimensions=1
  y : Outport  InitialOutput=0
  wires:
  u/1 -> FixPt Data Type Duplicate/2, FixPt Sum1/1
  FixPt Constant/1 -> sigspec/1
  FixPt Gateway In/1 -> FixPt Data Type Duplicate/3, FixPt Sum1/2
  FixPt Sum1/1 -> y/1, FixPt Data Type Duplicate/1
  sigspec/1 -> FixPt Gateway In/1

== system gm_UZ_EnDat/UZ_ENDAT/timingprovider/CLKCNTER_POSCNTR1/Positional_Counter/Increment Stored Integer ==
  u : Inport  OutDataTypeStr=uint32
  FixPt Constant : Constant  OutDataTypeStr=uint32  SampleTime=-1
  FixPt Data Type Duplicate : DataTypeDuplicate  DisableCoverage=on  NumInputPorts=3
  FixPt Gateway In : DataTypeConversion  OutDataTypeStr=fixdt(0,32,0)
  FixPt Sum1 : Sum  OutDataTypeStr=uint32  AccumDataTypeStr=uint32
  sigspec : SignalSpecification  OutDataTypeStr=uint32  Dimensions=1
  y : Outport  InitialOutput=0
  wires:
  FixPt Constant/1 -> sigspec/1
  FixPt Gateway In/1 -> FixPt Data Type Duplicate/3, FixPt Sum1/2
  FixPt Sum1/1 -> y/1, FixPt Data Type Duplicate/1
  sigspec/1 -> FixPt Gateway In/1
  u/1 -> FixPt Data Type Duplicate/2, FixPt Sum1/1
